simulink model "xpc8audiochannels"  (Simulink 6.0)
settings: Solver=FixedStepDiscrete  StartTime=0.0  StopTime=inf  RelTol=1e-3
libraries: xpclib x10, dspsigattribs x8
settings Model: Creator=gweast  LastModifiedBy=ekbas  ExtModeArmWhenConnect=off  BufferReuse=off  ProdHWDeviceType=Specified
settings DataIOCC: SignalLoggingName=sigsOut
settings OptimizationCC: BooleanDataType=off  InlineInvariantSignals=off  OptimizeBlockIOStorage=off  BufferReuse=off  EnforceIntegerDowncast=off  FoldNonRolledExpr=off  LocalBlockOutputs=off
settings DebuggingCC: CheckExecutionContextPreStartOutputMsg=on  CheckExecutionContextRuntimeOutputMsg=on  SolverPrmCheckMsg=none
settings HardwareCC: ProdHWDeviceType=Specified  TargetHWDeviceType=32-bit Generic  ProdEqTarget=off
settings RTWCC: SystemTargetFile=xpctarget.tlc  TemplateMakefile=xpc_default_tmf  ProcessScript=xpctarget_make_rtw_hook
settings xpcTargetCC: TargetFcnLib=ansi_tfl_tmw.mat  GenFloatMathFcnCalls=ANSI_C  ModelReferenceCompliant=off  LifeSpan=inf
settings SFSimCC: SFSimApplyToAllLibs=on  SFSimBuildMode=Incremental

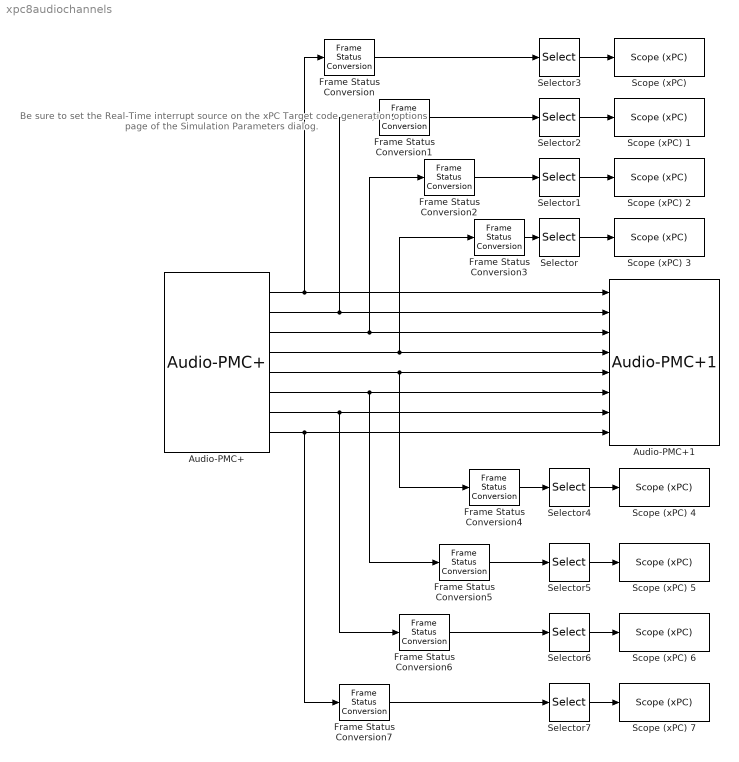
== system xpc8audiochannels ==
  note: Be sure to set the
      | Real-Time interrupt
      | source on the xPC Target
      | code generation options
      | page of the Simulation
      | Parameters dialog.
  Audio-PMC+ : xpclib/Audio/Bittware/Audio-PMC+  channel=[1 2 3 4 5 6 7 8]  framesize=64  samplerate=48000  convert=+-1.000  sampletime=-1  slot=-1
  Audio-PMC+1 : xpclib/Audio/Bittware/Audio-PMC+1  channel=[1 2 3 4 5 6 7 8]  framesize=64  samplerate=48000  sampletime=-1  slot=-1
  Frame Status Conversion{,1..7} (8 alike) : dspsigattribs/Frame Status Conversion  growRefPort=off  outframe=Sample-based
  "Scope (xPC) " : xpclib/Misc./Scope (xPC)   scopeno=1  scopetype=Target  autostart=on  viewmode=Graphical redraw  formatstr='%15.6f'  grid=on  ylimits=[0,0]  nosamples=500  noprepostsamples=0  interleave=1  triggermode=Signal triggering  triggersignal=1  triggerlevel=0.0  triggerslope=Rising  triggerscope=1  triggersample=0  filename=data.dat  mode=Lazy  writesize=512  autorestart=off
  Scope (xPC) 1 : xpclib/Misc./Scope (xPC)   scopeno=2  scopetype=Target  autostart=on  viewmode=Graphical redraw  formatstr='%15.6f'  grid=on  ylimits=[0,0]  nosamples=500  noprepostsamples=0  interleave=1  triggermode=Signal triggering  triggersignal=1  triggerlevel=0.0  triggerslope=Rising  triggerscope=1  triggersample=0  filename=data.dat  mode=Lazy  writesize=512  autorestart=off
  Scope (xPC) 2 : xpclib/Misc./Scope (xPC)   scopeno=3  scopetype=Target  autostart=on  viewmode=Graphical redraw  formatstr='%15.6f'  grid=on  ylimits=[0,0]  nosamples=500  noprepostsamples=0  interleave=1  triggermode=Signal triggering  triggersignal=1  triggerlevel=0.0  triggerslope=Rising  triggerscope=1  triggersample=0  filename=data.dat  mode=Lazy  writesize=512  autorestart=off
  Scope (xPC) 3 : xpclib/Misc./Scope (xPC)   scopeno=4  scopetype=Target  autostart=on  viewmode=Graphical redraw  formatstr='%15.6f'  grid=on  ylimits=[0,0]  nosamples=500  noprepostsamples=0  interleave=1  triggermode=Signal triggering  triggersignal=1  triggerlevel=0.0  triggerslope=Rising  triggerscope=1  triggersample=0  filename=data.dat  mode=Lazy  writesize=512  autorestart=off
  Scope (xPC) 4 : xpclib/Misc./Scope (xPC)   scopeno=5  scopetype=Target  autostart=on  viewmode=Graphical redraw  formatstr='%15.6f'  grid=on  ylimits=[0,0]  nosamples=500  noprepostsamples=0  interleave=1  triggermode=Signal triggering  triggersignal=1  triggerlevel=0.0  triggerslope=Rising  triggerscope=1  triggersample=0  filename=data.dat  mode=Lazy  writesize=512  autorestart=off
  Scope (xPC) 5 : xpclib/Misc./Scope (xPC)   scopeno=6  scopetype=Target  autostart=on  viewmode=Graphical redraw  formatstr='%15.6f'  grid=on  ylimits=[0,0]  nosamples=500  noprepostsamples=0  interleave=1  triggermode=Signal triggering  triggersignal=1  triggerlevel=0.0  triggerslope=Rising  triggerscope=1  triggersample=0  filename=data.dat  mode=Lazy  writesize=512  autorestart=off
  Scope (xPC) 6 : xpclib/Misc./Scope (xPC)   scopeno=7  scopetype=Target  autostart=on  viewmode=Graphical redraw  formatstr='%15.6f'  grid=on  ylimits=[0,0]  nosamples=500  noprepostsamples=0  interleave=1  triggermode=Signal triggering  triggersignal=1  triggerlevel=0.0  triggerslope=Rising  triggerscope=1  triggersample=0  filename=data.dat  mode=Lazy  writesize=512  autorestart=off
  Scope (xPC) 7 : xpclib/Misc./Scope (xPC)   scopeno=8  scopetype=Target  autostart=on  viewmode=Graphical redraw  formatstr='%15.6f'  grid=on  ylimits=[0,0]  nosamples=500  noprepostsamples=0  interleave=1  triggermode=Signal triggering  triggersignal=1  triggerlevel=0.0  triggerslope=Rising  triggerscope=1  triggersample=0  filename=data.dat  mode=Lazy  writesize=512  autorestart=off
  Selector{,1..7} (8 alike) : Selector  Elements=[1]
  wires:
  Audio-PMC+/1 -> Frame Status Conversion/1, Audio-PMC+1/1
  Audio-PMC+/2 -> Frame Status Conversion1/1, Audio-PMC+1/2
  Audio-PMC+/3 -> Frame Status Conversion2/1, Audio-PMC+1/3
  Audio-PMC+/4 -> Frame Status Conversion3/1, Audio-PMC+1/4
  Audio-PMC+/5 -> Frame Status Conversion4/1, Audio-PMC+1/5
  Audio-PMC+/6 -> Frame Status Conversion5/1, Audio-PMC+1/6
  Audio-PMC+/7 -> Frame Status Conversion6/1, Audio-PMC+1/7
  Audio-PMC+/8 -> Frame Status Conversion7/1, Audio-PMC+1/8
  Frame Status Conversion/1 -> Selector3/1
  Selector3/1 -> "Scope (xPC) "/1
  Frame Status Conversion1/1 -> Selector2/1
  Selector2/1 -> Scope (xPC) 1/1
  Frame Status Conversion2/1 -> Selector1/1
  Selector1/1 -> Scope (xPC) 2/1
  Frame Status Conversion3/1 -> Selector/1
  Selector/1 -> Scope (xPC) 3/1
  Frame Status Conversion4/1 -> Selector4/1
  Selector4/1 -> Scope (xPC) 4/1
  Frame Status Conversion5/1 -> Selector5/1
  Selector5/1 -> Scope (xPC) 5/1
  Frame Status Conversion6/1 -> Selector6/1
  Selector6/1 -> Scope (xPC) 6/1
  Frame Status Conversion7/1 -> Selector7/1
  Selector7/1 -> Scope (xPC) 7/1
